simulink library "GFM_Lib"  (R2021a)
settings: Solver=VariableStepAuto  StartTime=0.0  StopTime=10.0  RelTol=1e-3
values from neighbouring files (symbols this model uses):
  Lc_eq = Lc_pu + dLc_pu    [Init_VI_mmc.m]
  Lc_pu = Lt_pu+Larm_pu/2    [Init_VI_mmc.m]
  Rc_eq = Rc_pu    [Init_VI_mmc.m]
  Va0 = sqrt(2)*Vb1*Vvsc0*sin(Theta_vsc0*pi/180)    [Init_LF_LCL_old.m]
  Vb0 = sqrt(2)*Vb1*Vvsc0*sin(Theta_vsc0*pi/180-2*pi/3)    [Init_LF_LCL_old.m]
  Vc0 = sqrt(2)*Vb1*Vvsc0*sin(Theta_vsc0*pi/180+2*pi/3)    [Init_LF_LCL_old.m]
  Vm0_d = Vvsc0 * cos(Theta_vsc0*pi/180-Theta_m0*pi/180)    [Init_LF_LCL_old.m]
  Vm0_q = Vvsc0 * sin(Theta_vsc0*pi/180-Theta_m0*pi/180)    [Init_LF_LCL_old.m]
  Vvsc0 = abs(Vm)    [Init_LF_LCL_old.m]
undefined symbols (not defined in the file or in its folder): C_line, Carm, Cb, Delay_Equivalent, Delay_Flag, Diff_CC_ki, Diff_CC_kp, fb, Ib1, Ib2, Idcb, Ki_CC, Ki_Wdiff_pu, Ki_Wtot_pu, Kp_CC, Kp_Rvi_pu, Kp_Wdiff_pu, Kp_Wtot_pu, Lb, Sb, Tr_I_max, Vb1, Vb2, Vdcb, Vm0, VSC01_id0, wb, Zb
libraries: Control_Lib x88, spsVoltageMeasurementLib x26, spsSeriesRLCBranchLib x25, spsCurrentMeasurementLib x14, spsThreePhaseBreakerLib x12, spsThreePhaseSourceLib x12, spsThreePhaseVIMeasurementLib x12, spsControlledCurrentSourceLib x12, spsControlledVoltageSourceLib x12, simulink x11, spsSecondOrderFilterLib x8, spsUniversalBridgeLib x6
(part 6 of 6)

== system GFM_Lib/GFM_VC MMC/Control loops/DC part: stored energy control + differential current control/Control Wtot  ==
  note: Reference of i_diff --> adjusting dc power
  note: Energy based control
      |
      | dW
      | ----- = Pdc - Pac --> In this simulation, the energy is regulated by adjusting dc power
      | dt
      |
      | Pdc = PIcontroller*(W_ref - W_mes) + Pac
  note: ac power is considered as a disturbance
  Wtot_pu : Inport
  Wtot ref pu : Inport  Port=2
  p_ac_pu : Inport  Port=3
  Vdc_pu : Inport  Port=4
  Divide1 : Product  Inputs=/*
  Gain : Gain  Gain=-1
  Gain1 : Gain  Gain=1/3
  Gain_i 1 : Gain  Gain=Kp_Wtot_pu  SaturateOnIntegerOverflow=on  OutDataTypeStr=Inherit: Same as input  ParamDataTypeStr=Inherit: Same as input
  Gain_i 5 : Gain  Gain=Ki_Wtot_pu  SaturateOnIntegerOverflow=on  OutDataTypeStr=Inherit: Same as input  ParamDataTypeStr=Inherit: Same as input
  Integrator : Integrator  InitialConditionSource=external
  Sum : Sum  Inputs=++|
  Sum1 : Sum  InputSameDT=on  SaturateOnIntegerOverflow=on  OutDataTypeStr=Inherit: Same as first input
  Sum4 : Sum  Inputs=+-  InputSameDT=on  SaturateOnIntegerOverflow=on  OutDataTypeStr=Inherit: Same as first input
  Idiff ref pu : Outport
  wires:
  Gain/1 -> Integrator/2
  Sum/1 -> Divide1/2
  Divide1/1 -> Idiff ref pu/1  "idiff_ref"
  Vdc_pu/1 -> Divide1/1
  Sum1/1 -> Sum/2
  Sum4/1 -> Gain_i 1/1, Gain_i 5/1
  Gain_i 5/1 -> Integrator/1
  Integrator/1 -> Sum1/1
  Gain_i 1/1 -> Sum1/2, Gain/1
  Wtot ref pu/1 -> Sum4/1
  Wtot_pu/1 -> Sum4/2
  p_ac_pu/1 -> Gain1/1
  Gain1/1 -> Sum/1

== system GFM_Lib/GFM_VC MMC/Control loops/DC part: stored energy control + differential current control/Differential_current_control ==
  vdc_pu : Inport
  idiff_pu : Inport  Port=2
  idiff_ref_pu : Inport  Port=3
  Constant : Constant
  Gain3 : Gain  Gain=1/2
  Gain_i 1 : Gain  Gain=Diff_CC_kp  SaturateOnIntegerOverflow=on  OutDataTypeStr=Inherit: Same as input  ParamDataTypeStr=Inherit: Same as input
  Gain_i 5 : Gain  Gain=Diff_CC_ki  SaturateOnIntegerOverflow=on  OutDataTypeStr=Inherit: Same as input  ParamDataTypeStr=Inherit: Same as input
  Integrator : Integrator
  Scope : Scope  NumInputPorts=2
  Sum1 : Sum  Inputs=+-  InputSameDT=on  SaturateOnIntegerOverflow=on  OutDataTypeStr=Inherit: Same as first input
  Sum2 : Sum  InputSameDT=on  SaturateOnIntegerOverflow=on  OutDataTypeStr=Inherit: Same as first input
  Sum3 : Sum  Inputs=+-  InputSameDT=on  SaturateOnIntegerOverflow=on  OutDataTypeStr=Inherit: Same as first input
  Vprediff_ref_pu : Outport
  wires:
  idiff_pu/1 -> Sum1/2, Scope/2
  idiff_ref_pu/1 -> Sum1/1, Scope/1
  Sum1/1 -> Gain_i 1/1, Gain_i 5/1
  Gain_i 5/1 -> Integrator/1
  Gain_i 1/1 -> Sum2/2
  Integrator/1 -> Sum2/1
  Constant/1 -> Gain3/1
  Gain3/1 -> Sum3/1
  Sum3/1 -> Vprediff_ref_pu/1
  Sum2/1 -> Sum3/2

== system GFM_Lib/GFM_VC MMC/Control loops/DC part: stored energy control + differential current control/Wdiff computation ==
  vctot u_pu : Inport
  vctot l_pu : Inport  Port=2
  Gain10 : Gain  Gain=1/2
  Moving Average1 : eeGeneralControl/Moving Average  Commented=on  VariantControl=Variant1  LabelModeActiveChoice=Discrete  f=50  x0=0  Ts=-1
      settings: SourceProductBaseCode=PS
  Product : Product
  Product1 : Product
  Second-Order Filter1 : spsSecondOrderFilterLib/Second-Order Filter  FilterType=Bandstop (Notch)  Fo=fb  Zeta=1  Ts=0  Initialize=on  Vac_Init="[0,  0,  60; 0, 0, 60; 0, 0, 60]"  Vdc_Init=[0, 0, 0]  PlotResponse=off  FreqRange=[0, 500, 1]
      settings: SourceProductBaseCode=PS
  Sum3 : Sum  Inputs=+-
  Wdiff : Outport  PortDimensions=3
  wires:
  vctot u_pu/1 -> Product/2, Product/1
  Sum3/1 -> Gain10/1
  vctot l_pu/1 -> Product1/2, Product1/1
  Product/1 -> Sum3/1
  Product1/1 -> Sum3/2
  Second-Order Filter1/1 -> Wdiff/1
  Gain10/1 -> Second-Order Filter1/1

== system GFM_Lib/GFM_VC MMC/Control loops/DC part: stored energy control + differential current control/Wtot computation ==
  vctot u_pu : Inport
  vctot l_pu : Inport  Port=2
  Gain10 : Gain  Gain=1/2
  Moving Average1 : eeGeneralControl/Moving Average  Commented=on  VariantControl=Variant1  LabelModeActiveChoice=Discrete  f=50  x0=1  Ts=-1
      settings: SourceProductBaseCode=PS
  Product : Product
  Product1 : Product
  Second-Order Filter : spsSecondOrderFilterLib/Second-Order Filter  FilterType=Bandstop (Notch)  Fo=2*fb  Zeta=1  Ts=0  Initialize=on  Vac_Init="[0,  0,  60; 0, 0, 60; 0, 0, 60]"  Vdc_Init=[1; 1; 1]  PlotResponse=off  FreqRange=[0, 500, 1]
      settings: SourceProductBaseCode=PS
  Sum3 : Sum
  Wtot : Outport  PortDimensions=3
  wires:
  vctot u_pu/1 -> Product/2, Product/1
  Sum3/1 -> Gain10/1
  vctot l_pu/1 -> Product1/2, Product1/1
  Product/1 -> Sum3/1
  Product1/1 -> Sum3/2
  Second-Order Filter/1 -> Wtot/1
  Gain10/1 -> Second-Order Filter/1

== system GFM_Lib/GFM_VC MMC/Control loops/TVI/dq to phasor ==
  dq_mes : Inport
  Demux : Demux  Outputs=2
      settings: DisplayOption=none
  Sqrt : Sqrt  SaturateOnIntegerOverflow=on
  Sum4 : Sum  Inputs=|++  InputSameDT=on  SaturateOnIntegerOverflow=on  OutDataTypeStr=Inherit: Same as first input
  Vrdird : Product  InputSameDT=on  RndMeth=Zero  SaturateOnIntegerOverflow=on  OutDataTypeStr=Inherit: Same as first input
  Vrqirq : Product  InputSameDT=on  RndMeth=Zero  SaturateOnIntegerOverflow=on  OutDataTypeStr=Inherit: Same as first input
  rms : Outport  VectorParamsAs1DForOutWhenUnconnected=off
  wires:
  Sum4/1 -> Sqrt/1
  Vrqirq/1 -> Sum4/2
  Vrdird/1 -> Sum4/1
  Demux/2 -> Vrqirq/2, Vrqirq/1
  Demux/1 -> Vrdird/2, Vrdird/1
  dq_mes/1 -> Demux/1
  Sqrt/1 -> rms/1

== system GFM_Lib/GFM_VC MMC/Control loops/Transient Damping Resistance/Filter w_LF ==
  e : Inport
  1/T_LP : Gain  Gain=W_TVR  SaturateOnIntegerOverflow=on  OutDataTypeStr=Inherit: Same as input  ParamDataTypeStr=Inherit: Same as input
  Integrator : Integrator  InitialConditionSource=external  InitialCondition=[VSC01_id0*0.04]
  Sum1 : Sum  Inputs=|+-  InputSameDT=on  SaturateOnIntegerOverflow=on  OutDataTypeStr=Inherit: Same as first input
  s : Outport  VectorParamsAs1DForOutWhenUnconnected=off
  wires:
  e/1 -> Sum1/1, Integrator/2
  Integrator/1 -> s/1, Sum1/2
  1/T_LP/1 -> Integrator/1
  Sum1/1 -> 1/T_LP/1

== system GFM_Lib/GFM_CC IDEAL_VSC/Control loops/Current control/Current control/LPF1 ==
  In1 : Inport
  Add : Sum  Inputs=+-
  Gain : Gain  Gain=w_ff
  Integrator : Integrator  InitialCondition=V0*cos(Theta0*pi/180)
  Out1 : Outport
  wires:
  Add/1 -> Gain/1
  Gain/1 -> Integrator/1
  Integrator/1 -> Out1/1, Add/2
  In1/1 -> Add/1

== system GFM_Lib/GFM_CC IDEAL_VSC/Control loops/Current control/Current control/LPF2 ==
  In1 : Inport
  Add : Sum  Inputs=+-
  Gain : Gain  Gain=w_ff
  Integrator : Integrator  InitialCondition=V0*sin(Theta0*pi/180)
  Out1 : Outport
  wires:
  Add/1 -> Gain/1
  Gain/1 -> Integrator/1
  Integrator/1 -> Out1/1, Add/2
  In1/1 -> Add/1

== system GFM_Lib/GFM_CC LCL_FILTER_VSC/Control loops/Inner Cascaded control loops/Current Limitation/Current control ==
  Ig_dq0* : Inport
  Ig_dq0 : Inport  Port=2
  vg_dq0 : Inport  Port=3
  w : Inport  Port=4
  Demux : Demux  Outputs=2
  Demux1 : Demux  Outputs=2
  Demux2 : Demux  Outputs=2
  Gain Corrector : Gain  Gain=wn_I_max*Lt_pu
  Gain Corrector1 : Gain  Gain=wn_I_max*Lt_pu
  Mux : Mux  Inputs=2
  Product : Product  RndMeth=Zero
  Product1 : Product  RndMeth=Zero
  Sum : Sum  Inputs=|+-
  Sum2 : Sum  Inputs=|+-
  Sum3 : Sum  Inputs=|++
  Sum5 : Sum  Inputs=++|
  Sum6 : Sum  Inputs=-+|
  Sum7 : Sum  Inputs=++|
  w*Lf_pu : Gain  Gain=Lt_pu
  vm : Outport  InitialOutput=0  VectorParamsAs1DForOutWhenUnconnected=off
  wires:
  Demux2/2 -> Sum7/1
  Demux2/1 -> Sum3/2
  w/1 -> w*Lf_pu/1
  Sum/1 -> Gain Corrector/1
  Sum7/1 -> Mux/2  "Vm_q*"
  Sum3/1 -> Mux/1  "Vm_d*"
  Sum5/1 -> Sum7/2
  Product1/1 -> Sum5/1
  Gain Corrector1/1 -> Sum5/2
  Demux/2 -> Sum6/2
  Sum2/1 -> Sum3/1
  Product/1 -> Sum2/2
  Demux1/2 -> Sum6/1, Product/1
  w*Lf_pu/1 -> Product/2, Product1/1
  Gain Corrector/1 -> Sum2/1
  Demux1/1 -> Sum/2, Product1/2
  Demux/1 -> Sum/1
  Ig_dq0/1 -> Demux1/1
  vg_dq0/1 -> Demux2/1
  Sum6/1 -> Gain Corrector1/1
  Ig_dq0*/1 -> Demux/1
  Mux/1 -> vm/1

== system GFM_Lib/GFM_CC LCL_FILTER_VSC/Control loops/Inner Cascaded control loops/Current Limitation/Inverse Current control ==
  Vm_dq* : Inport
  Ig_dq : Inport  Port=2
  vg_dq : Inport  Port=3
  w : Inport  Port=4
  Demux : Demux  Outputs=2
  Demux1 : Demux  Outputs=2
  Demux2 : Demux  Outputs=2
  Gain Corrector2 : Gain  Gain=1/(wn_I_max*Lt_pu)
  Gain Corrector3 : Gain  Gain=1/(wn_I_max*Lt_pu)
  Mux : Mux  Inputs=2
  Product : Product  RndMeth=Zero
  Product1 : Product  RndMeth=Zero
  Sum : Sum  Inputs=|+-
  Sum2 : Sum  Inputs=|++
  Sum3 : Sum  Inputs=|++
  Sum5 : Sum  Inputs=-+|
  Sum6 : Sum  Inputs=-+|
  Sum7 : Sum  Inputs=++|
  w*Lf_pu : Gain  Gain=Lt_pu
  Is_dq* : Outport  InitialOutput=0  VectorParamsAs1DForOutWhenUnconnected=off
  wires:
  vg_dq/1 -> Demux2/1
  Ig_dq/1 -> Demux1/1
  Vm_dq*/1 -> Demux/1
  Demux/1 -> Sum/1
  Demux1/1 -> Sum3/2, Product1/2
  Sum/1 -> Sum2/1
  w*Lf_pu/1 -> Product1/1, Product/2
  Product/1 -> Sum2/2
  Sum2/1 -> Gain Corrector3/1
  Mux/1 -> Is_dq*/1
  Demux/2 -> Sum6/2
  Sum6/1 -> Sum5/2
  Sum5/1 -> Gain Corrector2/1
  Sum3/1 -> Mux/1  "is_d*"
  Sum7/1 -> Mux/2  "is_q*"
  w/1 -> w*Lf_pu/1
  Demux1/2 -> Sum7/1, Product/1
  Gain Corrector3/1 -> Sum3/1
  Demux2/1 -> Sum/2
  Demux2/2 -> Sum6/1
  Product1/1 -> Sum5/1
  Gain Corrector2/1 -> Sum7/2

== system GFM_Lib/GFM_CC MMC/Control loops/Current control/Current control/LPF1 ==
  In1 : Inport
  Add : Sum  Inputs=+-
  Gain : Gain  Gain=w_ff
  Integrator : Integrator  InitialCondition=V0*cos(Theta0*pi/180)
  Out1 : Outport
  wires:
  Add/1 -> Gain/1
  Gain/1 -> Integrator/1
  Integrator/1 -> Out1/1, Add/2
  In1/1 -> Add/1

== system GFM_Lib/GFM_CC MMC/Control loops/Current control/Current control/LPF2 ==
  In1 : Inport
  Add : Sum  Inputs=+-
  Gain : Gain  Gain=w_ff
  Integrator : Integrator  InitialCondition=V0*sin(Theta0*pi/180)
  Out1 : Outport
  wires:
  Add/1 -> Gain/1
  Gain/1 -> Integrator/1
  Integrator/1 -> Out1/1, Add/2
  In1/1 -> Add/1

== system GFM_Lib/GFM_VC LCL_FILTER_VSC/Control loops/Inner Cascaded control loops/Current Limitation/Current control ==
  Ig_dq0* : Inport
  Ig_dq0 : Inport  Port=2
  vg_dq0 : Inport  Port=3
  w : Inport  Port=4
  Demux : Demux  Outputs=2
  Demux1 : Demux  Outputs=2
  Demux2 : Demux  Outputs=2
  Gain Corrector : Gain  Gain=wn_I_max*Lt_pu/wb
  Gain Corrector1 : Gain  Gain=wn_I_max*Lt_pu/wb
  Mux : Mux  Inputs=2
  Product : Product  RndMeth=Zero
  Product1 : Product  RndMeth=Zero
  Sum : Sum  Inputs=|+-
  Sum2 : Sum  Inputs=|+-
  Sum3 : Sum  Inputs=|++
  Sum5 : Sum  Inputs=++|
  Sum6 : Sum  Inputs=-+|
  Sum7 : Sum  Inputs=++|
  w*Lf_pu : Gain  Gain=Lt_pu
  vm : Outport  InitialOutput=0  VectorParamsAs1DForOutWhenUnconnected=off
  wires:
  Demux2/2 -> Sum7/1
  Demux2/1 -> Sum3/2
  w/1 -> w*Lf_pu/1
  Sum/1 -> Gain Corrector/1
  Sum7/1 -> Mux/2  "Vm_q*"
  Sum3/1 -> Mux/1  "Vm_d*"
  Sum5/1 -> Sum7/2
  Product1/1 -> Sum5/1
  Gain Corrector1/1 -> Sum5/2
  Demux/2 -> Sum6/2
  Sum2/1 -> Sum3/1
  Product/1 -> Sum2/2
  Demux1/2 -> Sum6/1, Product/1
  w*Lf_pu/1 -> Product/2, Product1/1
  Gain Corrector/1 -> Sum2/1
  Demux1/1 -> Sum/2, Product1/2
  Demux/1 -> Sum/1
  Ig_dq0/1 -> Demux1/1
  vg_dq0/1 -> Demux2/1
  Sum6/1 -> Gain Corrector1/1
  Ig_dq0*/1 -> Demux/1
  Mux/1 -> vm/1

== system GFM_Lib/GFM_VC LCL_FILTER_VSC/Control loops/Inner Cascaded control loops/Current Limitation/Inverse Current control ==
  Vm_dq* : Inport
  Ig_dq : Inport  Port=2
  vg_dq : Inport  Port=3
  w : Inport  Port=4
  Demux : Demux  Outputs=2
  Demux1 : Demux  Outputs=2
  Demux2 : Demux  Outputs=2
  Gain Corrector2 : Gain  Gain=1/(wn_I_max*Lt_pu/wb)
  Gain Corrector3 : Gain  Gain=1/(wn_I_max*Lt_pu/wb)
  Mux : Mux  Inputs=2
  Product : Product  RndMeth=Zero
  Product1 : Product  RndMeth=Zero
  Sum : Sum  Inputs=|+-
  Sum2 : Sum  Inputs=|++
  Sum3 : Sum  Inputs=|++
  Sum5 : Sum  Inputs=-+|
  Sum6 : Sum  Inputs=-+|
  Sum7 : Sum  Inputs=++|
  w*Lf_pu : Gain  Gain=Lt_pu
  Is_dq* : Outport  InitialOutput=0  VectorParamsAs1DForOutWhenUnconnected=off
  wires:
  vg_dq/1 -> Demux2/1
  Ig_dq/1 -> Demux1/1
  Vm_dq*/1 -> Demux/1
  Demux/1 -> Sum/1
  Demux1/1 -> Sum3/2, Product1/2
  Sum/1 -> Sum2/1
  w*Lf_pu/1 -> Product1/1, Product/2
  Product/1 -> Sum2/2
  Sum2/1 -> Gain Corrector3/1
  Mux/1 -> Is_dq*/1
  Demux/2 -> Sum6/2
  Sum6/1 -> Sum5/2
  Sum5/1 -> Gain Corrector2/1
  Sum3/1 -> Mux/1  "is_d*"
  Sum7/1 -> Mux/2  "is_q*"
  w/1 -> w*Lf_pu/1
  Demux1/2 -> Sum7/1, Product/1
  Gain Corrector3/1 -> Sum3/1
  Demux2/1 -> Sum/2
  Demux2/2 -> Sum6/1
  Product1/1 -> Sum5/1
  Gain Corrector2/1 -> Sum7/2
